simulink model "KinematicModel2"  (R2025a)
settings: Solver=FixedStepAuto  StartTime=0.0  StopTime=10.0  RelTol=1e-3
undefined symbols (not defined in the file): c
settings Model: DataDictionary=Constants.sldd  Creator=levirogalla  LastModifiedBy=levirogalla

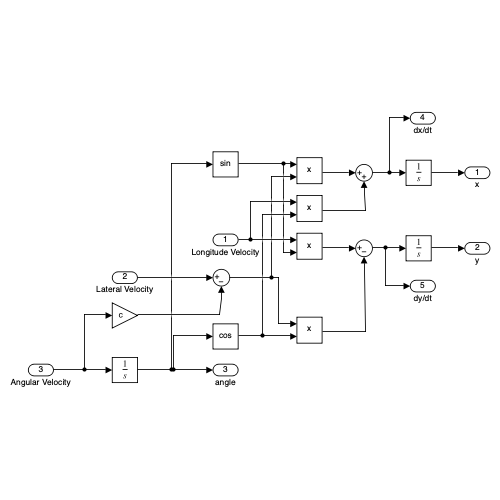
[thumbnail: Simulink's stored preview of the top-level diagram]
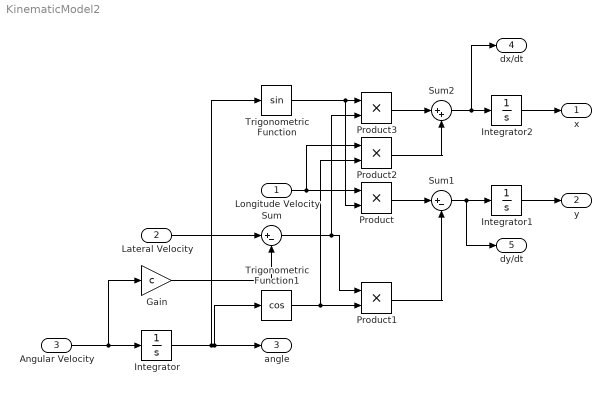
== system KinematicModel2 ==
  Longitude Velocity : Inport
  Lateral Velocity : Inport  Port=2
  Angular Velocity : Inport  Port=3
  Gain : Gain  Gain=c
  Integrator : Integrator
  Integrator1 : Integrator
  Integrator2 : Integrator
  Product{,1..3} (4 alike) : Product
  Sum : Sum  Inputs=|+-
  Sum1 : Sum  Inputs=|+-
  Sum2 : Sum  Inputs=|++
  Trigonometric Function : Trigonometry
  Trigonometric Function1 : Trigonometry  Operator=cos
  x : Outport
  y : Outport  Port=2
  angle : Outport  Port=3
  dx/dt : Outport  Port=4
  dy/dt : Outport  Port=5
  wires:
  Integrator1/1 -> y/1
  Integrator2/1 -> x/1
  Sum2/1 -> dx/dt/1, Integrator2/1
  Sum/1 -> Product3/2, Product1/1
  Product/1 -> Sum1/1
  Trigonometric Function1/1 -> Product2/2, Product1/2
  Product1/1 -> Sum1/2
  Longitude Velocity/1 -> Product2/1, Product/1
  Trigonometric Function/1 -> Product3/1, Product/2
  Integrator/1 -> angle/1, Trigonometric Function1/1, Trigonometric Function/1
  Product3/1 -> Sum2/1
  Lateral Velocity/1 -> Sum/1
  Sum1/1 -> dy/dt/1, Integrator1/1
  Product2/1 -> Sum2/2
  Gain/1 -> Sum/2
  Angular Velocity/1 -> Gain/1, Integrator/1
